simulink model "BicycleModel"  (R2018b)
settings: Solver=ode1  StartTime=0.0  StopTime=10.0  FixedStep=0.001  RelTol=1e-3
undefined symbols (not defined in the file): env, sim, vehicle
libraries: simulink x6
settings Model: Creator=ogihara  LastModifiedBy=ogihara

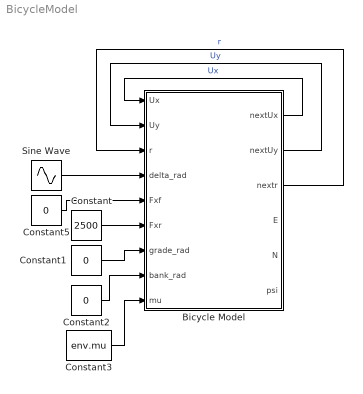
== system BicycleModel ==
  Bicycle Model : Subsystem
  Constant : Constant  Value=2500
  Constant1 : Constant  Value=0
  Constant2 : Constant  Value=0
  Constant3 : Constant  Value=env.mu
  Constant5 : Constant  Value=0
  Sine Wave : Sin  Amplitude=20/180*pi  Frequency=1.5  SampleTime=0
  wires:
  Constant/1 -> Bicycle Model/6(Fxr)
  Constant3/1 -> Bicycle Model/9(mu)
  Constant1/1 -> Bicycle Model/7(grade_rad)
  Constant2/1 -> Bicycle Model/8(bank_rad)
  Sine Wave/1 -> Bicycle Model/4(delta_rad)
  Bicycle Model/1(nextUx) -> Bicycle Model/1(Ux)  "Ux"
  Bicycle Model/2(nextUy) -> Bicycle Model/2(Uy)  "Uy"
  Bicycle Model/3(nextr) -> Bicycle Model/3(r)  "r"
  Constant5/1 -> Bicycle Model/5(Fxf)

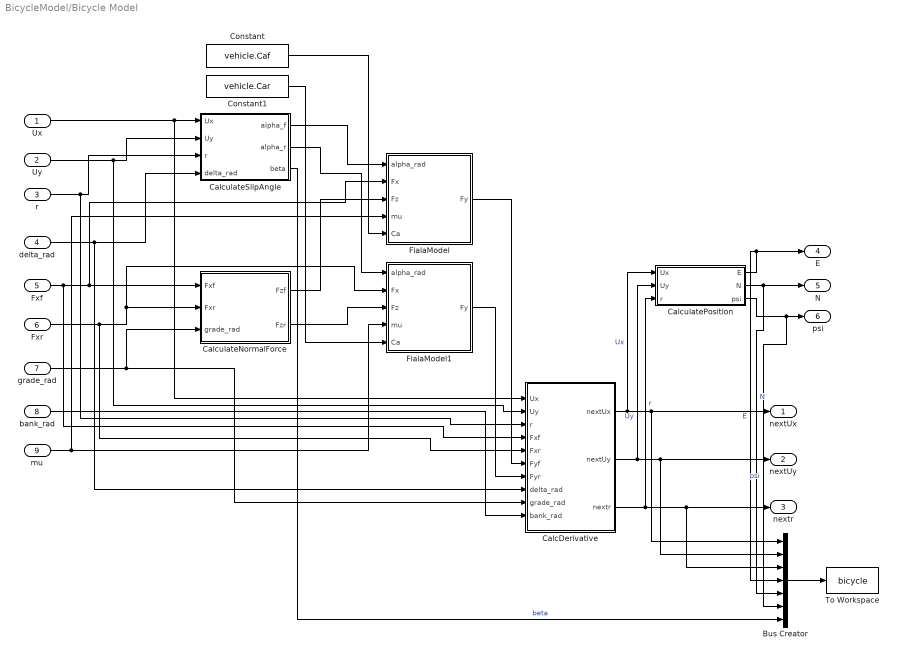
== system BicycleModel/Bicycle Model ==
  Ux : Inport
  Uy : Inport  Port=2
  r : Inport  Port=3
  delta_rad : Inport  Port=4
  Fxf : Inport  Port=5
  Fxr : Inport  Port=6
  grade_rad : Inport  Port=7
  bank_rad : Inport  Port=8
  mu : Inport  Port=9
  Bus Creator : BusCreator  Inputs=7
  CalcDerivative : Subsystem
  CalculateNormalForce : Subsystem
  CalculatePosition : Subsystem
  CalculateSlipAngle : Subsystem
  Constant : Constant  Value=vehicle.Caf
  Constant1 : Constant  Value=vehicle.Car
  FialaModel : Subsystem
  FialaModel1 : Subsystem
  To Workspace : ToWorkspace  VariableName=bicycle  SaveFormat=Timeseries  SampleTime=-1
  nextUx : Outport
  nextUy : Outport  Port=2
  nextr : Outport  Port=3
  E : Outport  Port=4
  N : Outport  Port=5
  psi : Outport  Port=6
  wires:
  Ux/1 -> CalcDerivative/1(Ux), CalculateSlipAngle/1(Ux)
  Uy/1 -> CalcDerivative/2(Uy), CalculateSlipAngle/2(Uy)
  r/1 -> CalcDerivative/3(r), CalculateSlipAngle/3(r)
  delta_rad/1 -> CalcDerivative/8(delta_rad), CalculateSlipAngle/4(delta_rad)
  Fxf/1 -> FialaModel/2(Fx), CalculateNormalForce/1(Fxf), CalcDerivative/4(Fxf)
  Fxr/1 -> FialaModel1/2(Fx), CalculateNormalForce/2(Fxr), CalcDerivative/5(Fxr)
  grade_rad/1 -> CalcDerivative/9(grade_rad), CalculateNormalForce/3(grade_rad)
  bank_rad/1 -> CalcDerivative/10(bank_rad)
  CalculateSlipAngle/1(alpha_f) -> FialaModel/1(alpha_rad)
  CalculateSlipAngle/2(alpha_r) -> FialaModel1/1(alpha_rad)
  CalculateNormalForce/1(Fzf) -> FialaModel/3(Fz)
  mu/1 -> FialaModel1/4(mu), FialaModel/4(mu)
  Constant1/1 -> FialaModel1/5(Ca)
  Constant/1 -> FialaModel/5(Ca)
  CalculateNormalForce/2(Fzr) -> FialaModel1/3(Fz)
  FialaModel/1(Fy) -> CalcDerivative/6(Fyf)
  FialaModel1/1(Fy) -> CalcDerivative/7(Fyr)
  CalculatePosition/1(E) -> E/1, Bus Creator/4  "E"
  CalculatePosition/2(N) -> N/1, Bus Creator/5  "N"
  Bus Creator/1 -> To Workspace/1
  CalcDerivative/3(nextr) -> CalculatePosition/3(r), Bus Creator/3, nextr/1  "r"
  CalcDerivative/1("nextUx ") -> CalculatePosition/1(Ux), nextUx/1, Bus Creator/1  "Ux"
  CalcDerivative/2(nextUy) -> nextUy/1, Bus Creator/2, CalculatePosition/2(Uy)  "Uy"
  CalculatePosition/3(psi) -> Bus Creator/6, psi/1  "psi"
  CalculateSlipAngle/3(beta) -> Bus Creator/7  "beta"

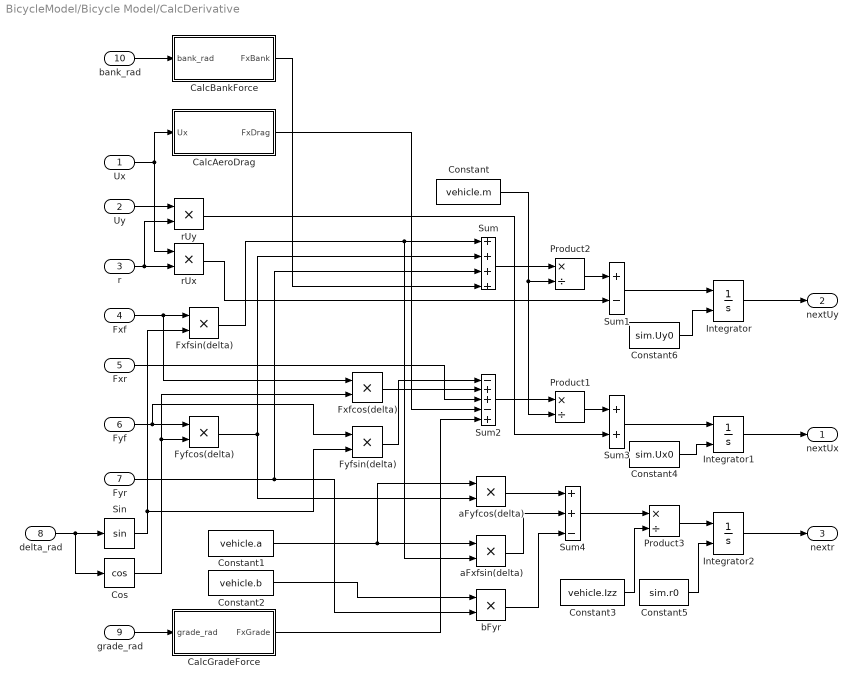
== system BicycleModel/Bicycle Model/CalcDerivative ==
  Ux : Inport
  Uy : Inport  Port=2
  r : Inport  Port=3
  Fxf : Inport  Port=4
  Fxr : Inport  Port=5
  Fyf : Inport  Port=6
  Fyr : Inport  Port=7
  delta_rad : Inport  Port=8
  grade_rad : Inport  Port=9
  bank_rad : Inport  Port=10
  CalcAeroDrag : Subsystem
  CalcBankForce : Subsystem
  CalcGradeForce : Subsystem
  Constant : Constant  Value=vehicle.m
  Constant1 : Constant  Value=vehicle.a
  Constant2 : Constant  Value=vehicle.b
  Constant3 : Constant  Value=vehicle.Izz
  Constant4 : Constant  Value=sim.Ux0
  Constant5 : Constant  Value=sim.r0
  Constant6 : Constant  Value=sim.Uy0
  Cos : Trigonometry  Operator=cos
  Fxfcos(delta) : Product
  Fxfsin(delta) : Product
  Fyfcos(delta) : Product
  Fyfsin(delta) : Product
  Integrator : Integrator  InitialConditionSource=external
  Integrator1 : Integrator  InitialConditionSource=external
  Integrator2 : Integrator  InitialConditionSource=external  InitialCondition=sim.r0
  Product1 : Product  Inputs=*/
  Product2 : Product  Inputs=*/
  Product3 : Product  Inputs=*/
  Sin : Trigonometry
  Sum : Sum  Inputs=++++
  Sum1 : Sum  Inputs=+-
  Sum2 : Sum  Inputs=-++-+
  Sum3 : Sum
  Sum4 : Sum  Inputs=++-
  aFxfsin(delta) : Product
  aFyfcos(delta) : Product
  bFyr : Product
  rUx : Product
  rUy : Product
  "nextUx " : Outport
  nextUy : Outport  Port=2
  nextr : Outport  Port=3
  wires:
  delta_rad/1 -> Cos/1, Sin/1
  Fyf/1 -> Fyfsin(delta)/1, Fyfcos(delta)/1
  Cos/1 -> Fxfcos(delta)/2, Fyfcos(delta)/2
  Fxf/1 -> Fxfcos(delta)/1, Fxfsin(delta)/1
  Sin/1 -> Fyfsin(delta)/2, Fxfsin(delta)/2
  Fxfsin(delta)/1 -> Sum/1, aFxfsin(delta)/2
  Fyfcos(delta)/1 -> aFyfcos(delta)/2, Sum/2
  Fyr/1 -> bFyr/2, Sum/3
  grade_rad/1 -> CalcGradeForce/1(grade_rad)
  Constant/1 -> Product1/2, Product2/2
  Sum/1 -> Product2/1
  r/1 -> rUx/2, rUy/2
  Ux/1 -> CalcAeroDrag/1(Ux), rUx/1
  Product2/1 -> Sum1/1
  Sum1/1 -> Integrator/1
  rUx/1 -> Sum1/2
  Uy/1 -> rUy/1
  bank_rad/1 -> CalcBankForce/1(bank_rad)
  CalcBankForce/1(FxBank) -> Sum/4
  Fxr/1 -> Sum2/3
  CalcAeroDrag/1(FxDrag) -> Sum2/4
  CalcGradeForce/1(FxGrade) -> Sum2/5
  Product1/1 -> Sum3/1
  Sum2/1 -> Product1/1
  rUy/1 -> Sum3/2
  Constant1/1 -> aFxfsin(delta)/1, aFyfcos(delta)/1
  Constant2/1 -> bFyr/1
  aFyfcos(delta)/1 -> Sum4/1
  aFxfsin(delta)/1 -> Sum4/2
  bFyr/1 -> Sum4/3
  Constant3/1 -> Product3/2
  Sum4/1 -> Product3/1
  Product3/1 -> Integrator2/1
  Integrator/1 -> nextUy/1
  Integrator1/1 -> "nextUx "/1
  Integrator2/1 -> nextr/1
  Fyfsin(delta)/1 -> Sum2/1
  Fxfcos(delta)/1 -> Sum2/2
  Constant4/1 -> Integrator1/2
  Constant6/1 -> Integrator/2
  Sum3/1 -> Integrator1/1
  Constant5/1 -> Integrator2/2

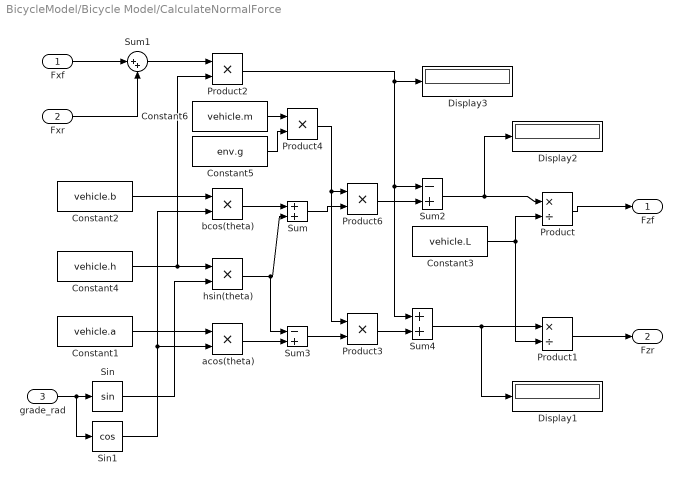
== system BicycleModel/Bicycle Model/CalculateNormalForce ==
  Fxf : Inport
  Fxr : Inport  Port=2
  grade_rad : Inport  Port=3
  Constant1 : Constant  Value=vehicle.a
  Constant2 : Constant  Value=vehicle.b
  Constant3 : Constant  Value=vehicle.L
  Constant4 : Constant  Value=vehicle.h
  Constant5 : Constant  Value=env.g
  Constant6 : Constant  Value=vehicle.m
  Display1 : Display
  Display2 : Display
  Display3 : Display
  Product : Product  Inputs=*/
  Product1 : Product  Inputs=*/
  Product{2..4,6} (4 alike) : Product
  Sin : Trigonometry
  Sin1 : Trigonometry  Operator=cos
  Sum : Sum
  Sum1 : Sum  Inputs=|++
  Sum2 : Sum  Inputs=-+
  Sum3 : Sum  Inputs=-+
  Sum4 : Sum
  acos(theta) : Product
  bcos(theta) : Product
  hsin(theta) : Product
  Fzf : Outport
  Fzr : Outport  Port=2
  wires:
  grade_rad/1 -> Sin1/1, Sin/1
  Constant2/1 -> bcos(theta)/1
  Sin1/1 -> bcos(theta)/2, acos(theta)/2
  Constant1/1 -> acos(theta)/1
  Sin/1 -> hsin(theta)/2
  bcos(theta)/1 -> Sum/1
  hsin(theta)/1 -> Sum3/1, Sum/2
  Sum/1 -> Product6/2
  Fxf/1 -> Sum1/1
  Fxr/1 -> Sum1/2
  Constant4/1 -> Product2/2, hsin(theta)/1
  Sum1/1 -> Product2/1
  Product6/1 -> Sum2/2
  Product2/1 -> Display3/1, Sum4/1, Sum2/1
  Sum2/1 -> Display2/1, Product/1
  Product/1 -> Fzf/1
  acos(theta)/1 -> Sum3/2
  Sum4/1 -> Display1/1, Product1/1
  Product3/1 -> Sum4/2
  Sum3/1 -> Product3/2
  Product1/1 -> Fzr/1
  Constant6/1 -> Product4/1
  Constant5/1 -> Product4/2
  Product4/1 -> Product3/1, Product6/1
  Constant3/1 -> Product1/2, Product/2

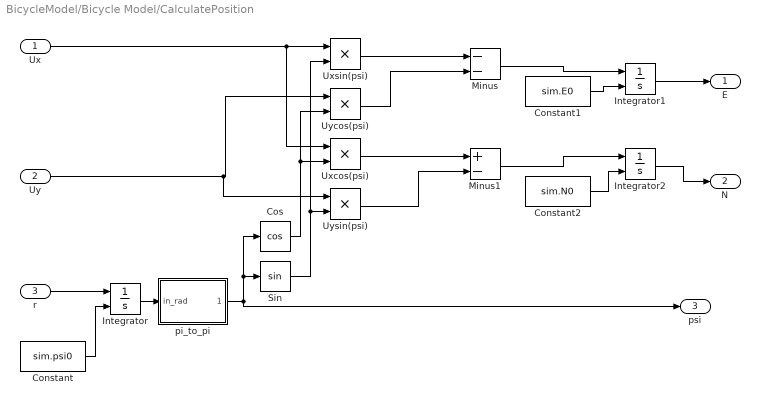
== system BicycleModel/Bicycle Model/CalculatePosition ==
  Ux : Inport
  Uy : Inport  Port=2
  r : Inport  Port=3
  Constant : Constant  Value=sim.psi0
  Constant1 : Constant  Value=sim.E0
  Constant2 : Constant  Value=sim.N0
  Cos : Trigonometry  Operator=cos
  Integrator : Integrator  InitialConditionSource=external
  Integrator1 : Integrator  InitialConditionSource=external
  Integrator2 : Integrator  InitialConditionSource=external
  Minus : Sum  Inputs=--
  Minus1 : Sum  Inputs=+-
  Sin : Trigonometry
  Uxcos(psi) : Product
  Uxsin(psi) : Product
  Uycos(psi) : Product
  Uysin(psi) : Product
  pi_to_pi : Subsystem
  E : Outport
  N : Outport  Port=2
  psi : Outport  Port=3
  wires:
  r/1 -> Integrator/1
  Constant/1 -> Integrator/2
  Integrator/1 -> pi_to_pi/1(in_rad)
  Integrator1/1 -> E/1
  Constant1/1 -> Integrator1/2
  Ux/1 -> Uxcos(psi)/1, Uxsin(psi)/1
  Sin/1 -> Uysin(psi)/2, Uxsin(psi)/2
  Uy/1 -> Uysin(psi)/1, Uycos(psi)/1
  Cos/1 -> Uxcos(psi)/2, Uycos(psi)/2
  Uxsin(psi)/1 -> Minus/1
  Uycos(psi)/1 -> Minus/2
  Minus/1 -> Integrator1/1
  Uxcos(psi)/1 -> Minus1/1
  Uysin(psi)/1 -> Minus1/2
  Minus1/1 -> Integrator2/1
  Constant2/1 -> Integrator2/2
  Integrator2/1 -> N/1
  pi_to_pi/1(out_rad) -> Sin/1, Cos/1, psi/1

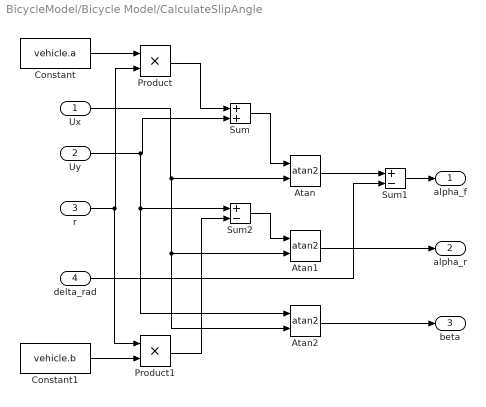
== system BicycleModel/Bicycle Model/CalculateSlipAngle ==
  Ux : Inport
  Uy : Inport  Port=2
  r : Inport  Port=3
  delta_rad : Inport  Port=4
  Atan : Trigonometry  Operator=atan2
  Atan1 : Trigonometry  Operator=atan2
  Atan2 : Trigonometry  Operator=atan2
  Constant : Constant  Value=vehicle.a
  Constant1 : Constant  Value=vehicle.b
  Product : Product
  Product1 : Product
  Sum : Sum
  Sum1 : Sum  Inputs=+-
  Sum2 : Sum  Inputs=+-
  alpha_f : Outport
  alpha_r : Outport  Port=2
  beta : Outport  Port=3
  wires:
  Constant/1 -> Product/1
  r/1 -> Product1/1, Product/2
  Constant1/1 -> Product1/2
  Ux/1 -> Atan2/2, Atan1/2, Atan/2
  Uy/1 -> Atan2/1, Sum2/1, Sum/2
  Product/1 -> Sum/1
  Sum/1 -> Atan/1
  delta_rad/1 -> Sum1/2
  Atan/1 -> Sum1/1
  Sum1/1 -> alpha_f/1
  Product1/1 -> Sum2/2
  Sum2/1 -> Atan1/1
  Atan1/1 -> alpha_r/1
  Atan2/1 -> beta/1

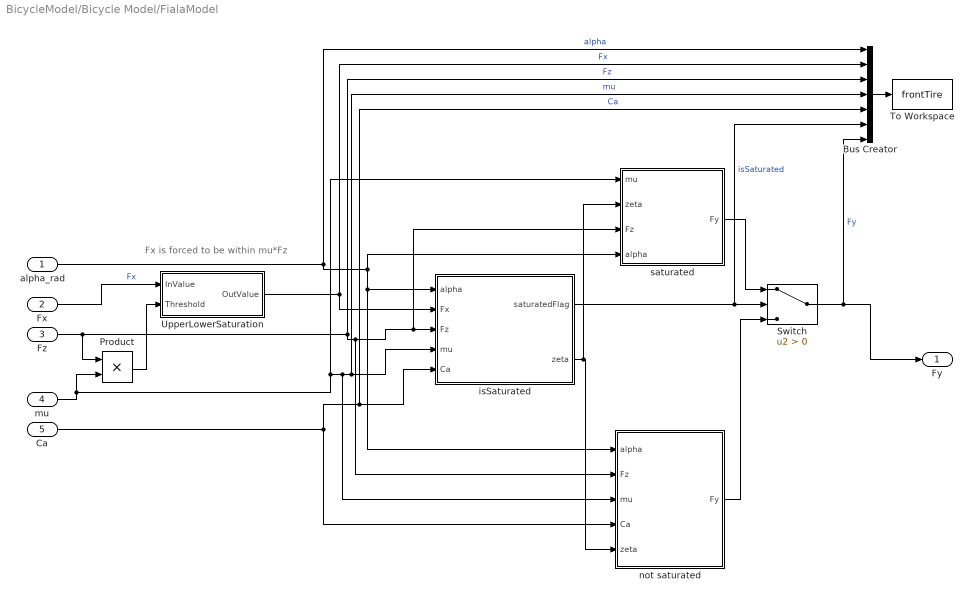
== system BicycleModel/Bicycle Model/FialaModel ==
  note: Fx is forced to be within mu*Fz
  alpha_rad : Inport
  Fx : Inport  Port=2
  Fz : Inport  Port=3
  mu : Inport  Port=4
  Ca : Inport  Port=5
  Bus Creator : BusCreator  Inputs=7
  Product : Product
  Switch : Switch  Criteria=u2 > Threshold
  To Workspace : ToWorkspace  VariableName=frontTire  SaveFormat=Timeseries  SampleTime=-1
  UpperLowerSaturation : Subsystem
  isSaturated : Subsystem
  not saturated : Subsystem
  saturated : Subsystem
  Fy : Outport
  wires:
  Switch/1 -> Bus Creator/7, Fy/1  "Fy"
  alpha_rad/1 -> not saturated/1(alpha), isSaturated/1(alpha), saturated/4(alpha), Bus Creator/1  "alpha"
  UpperLowerSaturation/1(OutValue) -> isSaturated/2(Fx), Bus Creator/2  "Fx"
  Fz/1 -> Product/1, not saturated/2(Fz), saturated/3(Fz), isSaturated/3(Fz), Bus Creator/3  "Fz"
  mu/1 -> Product/2, saturated/1(mu), not saturated/3(mu), Bus Creator/4, isSaturated/4(mu)  "mu"
  Ca/1 -> Bus Creator/5, isSaturated/5(Ca), not saturated/4(Ca)  "Ca"
  isSaturated/1(saturatedFlag) -> Bus Creator/6, Switch/2  "isSaturated"
  saturated/1(Fy) -> Switch/1
  not saturated/1(Fy) -> Switch/3
  isSaturated/2(zeta) -> saturated/2(zeta), not saturated/5(zeta)
  Bus Creator/1 -> To Workspace/1
  Fx/1 -> UpperLowerSaturation/1(InValue)  "Fx"
  Product/1 -> UpperLowerSaturation/2(Threshold)

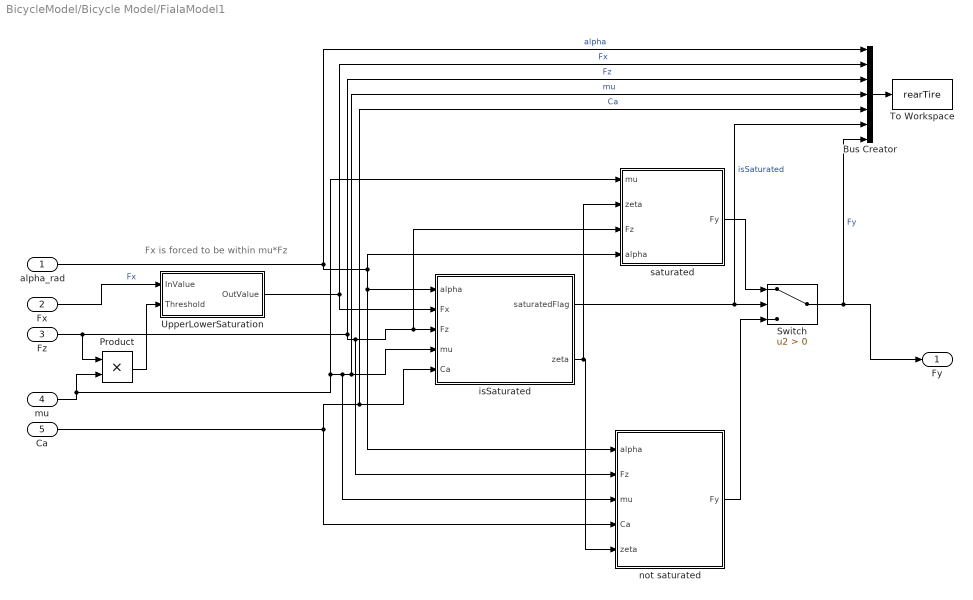
== system BicycleModel/Bicycle Model/FialaModel1 ==
  note: Fx is forced to be within mu*Fz
  alpha_rad : Inport
  Fx : Inport  Port=2
  Fz : Inport  Port=3
  mu : Inport  Port=4
  Ca : Inport  Port=5
  Bus Creator : BusCreator  Inputs=7
  Product : Product
  Switch : Switch  Criteria=u2 > Threshold
  To Workspace : ToWorkspace  VariableName=rearTire  SaveFormat=Timeseries  SampleTime=-1
  UpperLowerSaturation : Subsystem
  isSaturated : Subsystem
  not saturated : Subsystem
  saturated : Subsystem
  Fy : Outport
  wires:
  Switch/1 -> Bus Creator/7, Fy/1  "Fy"
  alpha_rad/1 -> not saturated/1(alpha), isSaturated/1(alpha), saturated/4(alpha), Bus Creator/1  "alpha"
  UpperLowerSaturation/1(OutValue) -> isSaturated/2(Fx), Bus Creator/2  "Fx"
  Fz/1 -> Product/1, not saturated/2(Fz), saturated/3(Fz), isSaturated/3(Fz), Bus Creator/3  "Fz"
  mu/1 -> Product/2, saturated/1(mu), not saturated/3(mu), Bus Creator/4, isSaturated/4(mu)  "mu"
  Ca/1 -> Bus Creator/5, isSaturated/5(Ca), not saturated/4(Ca)  "Ca"
  isSaturated/1(saturatedFlag) -> Bus Creator/6, Switch/2  "isSaturated"
  saturated/1(Fy) -> Switch/1
  not saturated/1(Fy) -> Switch/3
  isSaturated/2(zeta) -> saturated/2(zeta), not saturated/5(zeta)
  Bus Creator/1 -> To Workspace/1
  Fx/1 -> UpperLowerSaturation/1(InValue)  "Fx"
  Product/1 -> UpperLowerSaturation/2(Threshold)

== system BicycleModel/Bicycle Model/CalcDerivative/CalcAeroDrag ==
  Ux : Inport
  Constant : Constant  Value=vehicle.Cd0
  Gain : Gain  Gain=vehicle.Cd1
  Gain1 : Gain  Gain=vehicle.Cd2
  Product : Product
  Product1 : Product
  Sign : Signum
  Square : Math  Operator=square  SaturateOnIntegerOverflow=on
  Sum : Sum  Inputs=3
  FxDrag : Outport
  wires:
  Sum/1 -> FxDrag/1
  Gain1/1 -> Product1/2
  Gain/1 -> Sum/2
  Square/1 -> Gain1/1
  Ux/1 -> Gain/1, Square/1, Sign/1
  Product/1 -> Sum/1
  Sign/1 -> Product1/1, Product/2
  Constant/1 -> Product/1
  Product1/1 -> Sum/3

== system BicycleModel/Bicycle Model/CalcDerivative/CalcBankForce ==
  bank_rad : Inport
  Constant : Constant  Value=vehicle.m
  Constant1 : Constant  Value=env.g
  Product : Product  Inputs=3
  Sin : Trigonometry
  FxBank : Outport
  wires:
  bank_rad/1 -> Sin/1
  Sin/1 -> Product/1
  Constant/1 -> Product/2
  Constant1/1 -> Product/3
  Product/1 -> FxBank/1

== system BicycleModel/Bicycle Model/CalcDerivative/CalcGradeForce ==
  grade_rad : Inport
  Constant : Constant  Value=vehicle.m
  Constant1 : Constant  Value=env.g
  Product : Product  Inputs=3
  Sin : Trigonometry
  FxGrade : Outport
  wires:
  grade_rad/1 -> Sin/1
  Sin/1 -> Product/1
  Constant/1 -> Product/2
  Constant1/1 -> Product/3
  Product/1 -> FxGrade/1

== system BicycleModel/Bicycle Model/CalculatePosition/pi_to_pi ==
  in_rad : Inport
  Compare To Constant : simulink/Logic and Bit Operations/Compare To Constant  relop=<=  const=-pi  OutDataTypeStr=boolean
  Compare To Constant1 : simulink/Logic and Bit Operations/Compare To Constant  relop=>  const=pi  OutDataTypeStr=boolean
  Constant : Constant  Value=2*pi
  Minus : Sum  Inputs=+-
  Plus : Sum
  Switch : Switch  Criteria=u2 > Threshold
  Switch1 : Switch  Criteria=u2 > Threshold
  out_rad : Outport
  wires:
  Constant/1 -> Minus/2, Plus/2
  in_rad/1 -> Switch/3, Compare To Constant/1, Minus/1, Plus/1
  Compare To Constant1/1 -> Switch1/2
  Compare To Constant/1 -> Switch/2
  Plus/1 -> Switch/1
  Switch/1 -> Switch1/3, Compare To Constant1/1
  Minus/1 -> Switch1/1
  Switch1/1 -> out_rad/1

== system BicycleModel/Bicycle Model/FialaModel/UpperLowerSaturation ==
  note: Output is within [-Threshold, Threshold]
  InValue : Inport
  Threshold : Inport  Port=2
  Abs : Abs
  Gain : Gain  Gain=-1
  LowerSaturation : Subsystem
  UpperSaturation : Subsystem
  OutValue : Outport
  wires:
  LowerSaturation/1(OutVallue) -> OutValue/1
  Threshold/1 -> Abs/1
  InValue/1 -> UpperSaturation/1(InValue)
  Abs/1 -> Gain/1, UpperSaturation/2(Threshold)
  UpperSaturation/1(OutVallue) -> LowerSaturation/1(InValue)
  Gain/1 -> LowerSaturation/2(Threshold)

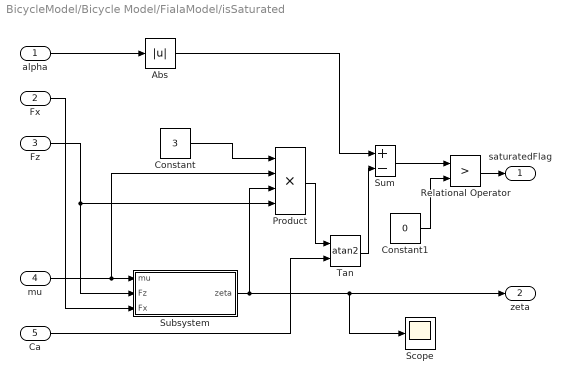
== system BicycleModel/Bicycle Model/FialaModel/isSaturated ==
  alpha : Inport
  Fx : Inport  Port=2
  Fz : Inport  Port=3
  mu : Inport  Port=4
  Ca : Inport  Port=5
  Abs : Abs
  Constant : Constant  Value=3
  Constant1 : Constant  Value=0
  Product : Product  Inputs=4
  Relational Operator : RelationalOperator  Operator=>  OutDataTypeStr=boolean  RndMeth=Simplest
  Scope : Scope
  Subsystem : Subsystem
  Sum : Sum  Inputs=+-
  Tan : Trigonometry  Operator=atan2
  saturatedFlag : Outport
  zeta : Outport  Port=2
  wires:
  Subsystem/1(zeta) -> Scope/1, zeta/1, Product/3
  Product/1 -> Tan/1
  Tan/1 -> Sum/2
  Fx/1 -> Subsystem/3(Fx)
  Fz/1 -> Subsystem/2(Fz), Product/4
  Constant/1 -> Product/1
  mu/1 -> Product/2, Subsystem/1(mu)
  Ca/1 -> Tan/2
  Abs/1 -> Sum/1
  alpha/1 -> Abs/1
  Sum/1 -> Relational Operator/1
  Constant1/1 -> Relational Operator/2
  Relational Operator/1 -> saturatedFlag/1

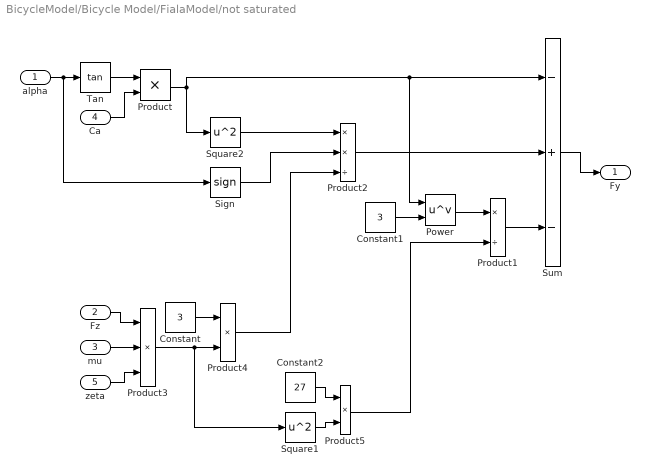
== system BicycleModel/Bicycle Model/FialaModel/not saturated ==
  alpha : Inport
  Fz : Inport  Port=2
  mu : Inport  Port=3
  Ca : Inport  Port=4
  zeta : Inport  Port=5
  Constant : Constant  Value=3
  Constant1 : Constant  Value=3
  Constant2 : Constant  Value=27
  Power : Math  Operator=pow  SaturateOnIntegerOverflow=on
  Product : Product
  Product1 : Product  Inputs=*/
  Product2 : Product  Inputs=**/
  Product3 : Product  Inputs=***
  Product4 : Product
  Product5 : Product
  Sign : Signum
  Square1 : Math  Operator=square  SaturateOnIntegerOverflow=on
  Square2 : Math  Operator=square  SaturateOnIntegerOverflow=on
  Sum : Sum  Inputs=-+-
  Tan : Trigonometry  Operator=tan
  Fy : Outport
  wires:
  Sum/1 -> Fy/1
  alpha/1 -> Sign/1, Tan/1
  Tan/1 -> Product/1
  Ca/1 -> Product/2
  Product/1 -> Square2/1, Power/1, Sum/1
  Square2/1 -> Product2/1
  Product2/1 -> Sum/2
  Fz/1 -> Product3/1
  mu/1 -> Product3/2
  zeta/1 -> Product3/3
  Product3/1 -> Square1/1, Product4/2
  Constant/1 -> Product4/1
  Product4/1 -> Product2/3
  Sign/1 -> Product2/2
  Constant2/1 -> Product5/1
  Square1/1 -> Product5/2
  Constant1/1 -> Power/2
  Power/1 -> Product1/1
  Product5/1 -> Product1/2
  Product1/1 -> Sum/3

== system BicycleModel/Bicycle Model/FialaModel/saturated ==
  mu : Inport
  zeta : Inport  Port=2
  Fz : Inport  Port=3
  alpha : Inport  Port=4
  Gain : Gain  Gain=-1
  Product : Product  Inputs=4
  Sign : Signum
  Fy : Outport
  wires:
  alpha/1 -> Sign/1
  Product/1 -> Gain/1
  Gain/1 -> Fy/1
  mu/1 -> Product/1
  zeta/1 -> Product/2
  Fz/1 -> Product/3
  Sign/1 -> Product/4

== system BicycleModel/Bicycle Model/FialaModel1/UpperLowerSaturation ==
  note: Output is within [-Threshold, Threshold]
  InValue : Inport
  Threshold : Inport  Port=2
  Abs : Abs
  Gain : Gain  Gain=-1
  LowerSaturation : Subsystem
  UpperSaturation : Subsystem
  OutValue : Outport
  wires:
  LowerSaturation/1(OutVallue) -> OutValue/1
  Threshold/1 -> Abs/1
  InValue/1 -> UpperSaturation/1(InValue)
  Abs/1 -> Gain/1, UpperSaturation/2(Threshold)
  UpperSaturation/1(OutVallue) -> LowerSaturation/1(InValue)
  Gain/1 -> LowerSaturation/2(Threshold)

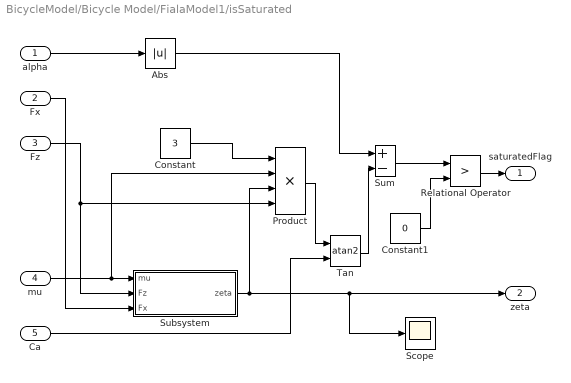
== system BicycleModel/Bicycle Model/FialaModel1/isSaturated ==
  alpha : Inport
  Fx : Inport  Port=2
  Fz : Inport  Port=3
  mu : Inport  Port=4
  Ca : Inport  Port=5
  Abs : Abs
  Constant : Constant  Value=3
  Constant1 : Constant  Value=0
  Product : Product  Inputs=4
  Relational Operator : RelationalOperator  Operator=>  OutDataTypeStr=boolean  RndMeth=Simplest
  Scope : Scope
  Subsystem : Subsystem
  Sum : Sum  Inputs=+-
  Tan : Trigonometry  Operator=atan2
  saturatedFlag : Outport
  zeta : Outport  Port=2
  wires:
  Subsystem/1(zeta) -> Scope/1, zeta/1, Product/3
  Product/1 -> Tan/1
  Tan/1 -> Sum/2
  Fx/1 -> Subsystem/3(Fx)
  Fz/1 -> Subsystem/2(Fz), Product/4
  Constant/1 -> Product/1
  mu/1 -> Product/2, Subsystem/1(mu)
  Ca/1 -> Tan/2
  Abs/1 -> Sum/1
  alpha/1 -> Abs/1
  Sum/1 -> Relational Operator/1
  Constant1/1 -> Relational Operator/2
  Relational Operator/1 -> saturatedFlag/1

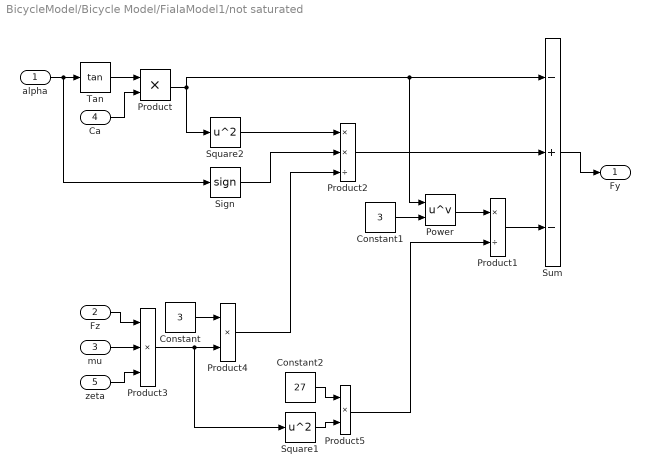
== system BicycleModel/Bicycle Model/FialaModel1/not saturated ==
  alpha : Inport
  Fz : Inport  Port=2
  mu : Inport  Port=3
  Ca : Inport  Port=4
  zeta : Inport  Port=5
  Constant : Constant  Value=3
  Constant1 : Constant  Value=3
  Constant2 : Constant  Value=27
  Power : Math  Operator=pow  SaturateOnIntegerOverflow=on
  Product : Product
  Product1 : Product  Inputs=*/
  Product2 : Product  Inputs=**/
  Product3 : Product  Inputs=***
  Product4 : Product
  Product5 : Product
  Sign : Signum
  Square1 : Math  Operator=square  SaturateOnIntegerOverflow=on
  Square2 : Math  Operator=square  SaturateOnIntegerOverflow=on
  Sum : Sum  Inputs=-+-
  Tan : Trigonometry  Operator=tan
  Fy : Outport
  wires:
  Sum/1 -> Fy/1
  alpha/1 -> Sign/1, Tan/1
  Tan/1 -> Product/1
  Ca/1 -> Product/2
  Product/1 -> Square2/1, Power/1, Sum/1
  Square2/1 -> Product2/1
  Product2/1 -> Sum/2
  Fz/1 -> Product3/1
  mu/1 -> Product3/2
  zeta/1 -> Product3/3
  Product3/1 -> Square1/1, Product4/2
  Constant/1 -> Product4/1
  Product4/1 -> Product2/3
  Sign/1 -> Product2/2
  Constant2/1 -> Product5/1
  Square1/1 -> Product5/2
  Constant1/1 -> Power/2
  Power/1 -> Product1/1
  Product5/1 -> Product1/2
  Product1/1 -> Sum/3

== system BicycleModel/Bicycle Model/FialaModel1/saturated ==
  mu : Inport
  zeta : Inport  Port=2
  Fz : Inport  Port=3
  alpha : Inport  Port=4
  Gain : Gain  Gain=-1
  Product : Product  Inputs=4
  Sign : Signum
  Fy : Outport
  wires:
  alpha/1 -> Sign/1
  Product/1 -> Gain/1
  Gain/1 -> Fy/1
  mu/1 -> Product/1
  zeta/1 -> Product/2
  Fz/1 -> Product/3
  Sign/1 -> Product/4

== system BicycleModel/Bicycle Model/FialaModel/UpperLowerSaturation/LowerSaturation ==
  note: If InValue is smaller than Threshold, Then OutValue is Threshold.
      | Else, OutValue is InValue.
  InValue : Inport
  Threshold : Inport  Port=2
  Compare To Zero : simulink/Logic and Bit Operations/Compare To Zero  relop=>  OutDataTypeStr=boolean
  Minus : Sum  Inputs=-+
  Switch : Switch  Criteria=u2 > Threshold
  OutVallue : Outport
  wires:
  Threshold/1 -> Switch/1, Minus/2
  InValue/1 -> Minus/1, Switch/3
  Minus/1 -> Compare To Zero/1
  Compare To Zero/1 -> Switch/2
  Switch/1 -> OutVallue/1

== system BicycleModel/Bicycle Model/FialaModel/UpperLowerSaturation/UpperSaturation ==
  note: If InValue is larger than Threshold, Then OutValue is Threshold.
      | Else, OutValue is InValue.
  InValue : Inport
  Threshold : Inport  Port=2
  Compare To Zero : simulink/Logic and Bit Operations/Compare To Zero  relop=>  OutDataTypeStr=boolean
  Minus : Sum  Inputs=+-
  Switch : Switch  Criteria=u2 > Threshold
  OutVallue : Outport
  wires:
  Threshold/1 -> Switch/1, Minus/2
  InValue/1 -> Switch/3, Minus/1
  Minus/1 -> Compare To Zero/1
  Compare To Zero/1 -> Switch/2
  Switch/1 -> OutVallue/1

== system BicycleModel/Bicycle Model/FialaModel/isSaturated/Subsystem ==
  mu : Inport
  Fz : Inport  Port=2
  Fx : Inport  Port=3
  Product : Product
  Product1 : Product  Inputs=*/
  Product2 : Product
  Sqrt : Sqrt  SaturateOnIntegerOverflow=on
  Square : Math  Operator=square  SaturateOnIntegerOverflow=on
  Square1 : Math  Operator=square  SaturateOnIntegerOverflow=on
  Square2 : Math  Operator=square  SaturateOnIntegerOverflow=on
  Sum : Sum  Inputs=+-
  zeta : Outport
  wires:
  mu/1 -> Product2/1, Square1/1
  Fz/1 -> Product2/2, Square/1
  Fx/1 -> Square2/1
  Square1/1 -> Product/1
  Square/1 -> Product/2
  Product/1 -> Sum/1
  Square2/1 -> Sum/2
  Sum/1 -> Sqrt/1
  Sqrt/1 -> Product1/1
  Product2/1 -> Product1/2
  Product1/1 -> zeta/1

== system BicycleModel/Bicycle Model/FialaModel1/UpperLowerSaturation/LowerSaturation ==
  note: If InValue is smaller than Threshold, Then OutValue is Threshold.
      | Else, OutValue is InValue.
  InValue : Inport
  Threshold : Inport  Port=2
  Compare To Zero : simulink/Logic and Bit Operations/Compare To Zero  relop=>  OutDataTypeStr=boolean
  Minus : Sum  Inputs=-+
  Switch : Switch  Criteria=u2 > Threshold
  OutVallue : Outport
  wires:
  Threshold/1 -> Switch/1, Minus/2
  InValue/1 -> Minus/1, Switch/3
  Minus/1 -> Compare To Zero/1
  Compare To Zero/1 -> Switch/2
  Switch/1 -> OutVallue/1

== system BicycleModel/Bicycle Model/FialaModel1/UpperLowerSaturation/UpperSaturation ==
  note: If InValue is larger than Threshold, Then OutValue is Threshold.
      | Else, OutValue is InValue.
  InValue : Inport
  Threshold : Inport  Port=2
  Compare To Zero : simulink/Logic and Bit Operations/Compare To Zero  relop=>  OutDataTypeStr=boolean
  Minus : Sum  Inputs=+-
  Switch : Switch  Criteria=u2 > Threshold
  OutVallue : Outport
  wires:
  Threshold/1 -> Switch/1, Minus/2
  InValue/1 -> Switch/3, Minus/1
  Minus/1 -> Compare To Zero/1
  Compare To Zero/1 -> Switch/2
  Switch/1 -> OutVallue/1

== system BicycleModel/Bicycle Model/FialaModel1/isSaturated/Subsystem ==
  mu : Inport
  Fz : Inport  Port=2
  Fx : Inport  Port=3
  Product : Product
  Product1 : Product  Inputs=*/
  Product2 : Product
  Sqrt : Sqrt  SaturateOnIntegerOverflow=on
  Square : Math  Operator=square  SaturateOnIntegerOverflow=on
  Square1 : Math  Operator=square  SaturateOnIntegerOverflow=on
  Square2 : Math  Operator=square  SaturateOnIntegerOverflow=on
  Sum : Sum  Inputs=+-
  zeta : Outport
  wires:
  mu/1 -> Product2/1, Square1/1
  Fz/1 -> Product2/2, Square/1
  Fx/1 -> Square2/1
  Square1/1 -> Product/1
  Square/1 -> Product/2
  Product/1 -> Sum/1
  Square2/1 -> Sum/2
  Sum/1 -> Sqrt/1
  Sqrt/1 -> Product1/1
  Product2/1 -> Product1/2
  Product1/1 -> zeta/1
